simulink model "simulink_431"  (R2024b)
settings: Solver=VariableStepAuto  StartTime=0.0  StopTime=10.0  RelTol=1e-3
values from neighbouring files (symbols this model uses):
  Cvp = cpp * rop * Vp    (= 75000)    [lab1_431.m]    (also in lab2_431.m)
  Cvw = cpp * rop * Vw    (= 300000)    [lab1_431.m]    (also in lab2_431.m)
  dPg = 1000    [lab1_431.m]    (also in lab2_431.m)
  dTzew = 0    [lab1_431.m]    (also in lab2_431.m)
  K1 = heatLossFactor * Kp    (= 240)    [lab1_431.m]    (also in lab2_431.m)
  Kd = Kp * (TwewN - TpN) / (TpN - TzewN)    (= 11.4285714286)    [lab1_431.m]    (also in lab2_431.m)
  Kp = PgN / (TwewN * (heatLossFactor + 1) - heatLossFactor * TzewN - TpN)    (= 80)    [lab1_431.m]    (also in lab2_431.m)
  Pg0 = workPoints(2, i)    [lab1_431.m]    (also in lab2_431.m = 7000)
  stepTime = 500    [lab1_431.m]    (also in lab2_431.m)
  Tzew0 = workPoints(1, i)    [lab1_431.m]    (also in lab2_431.m = -20)
undefined symbols (not defined in the file or in its folder): Tp0, Twew0
settings Model: Creator=maria  LastModifiedBy=maria

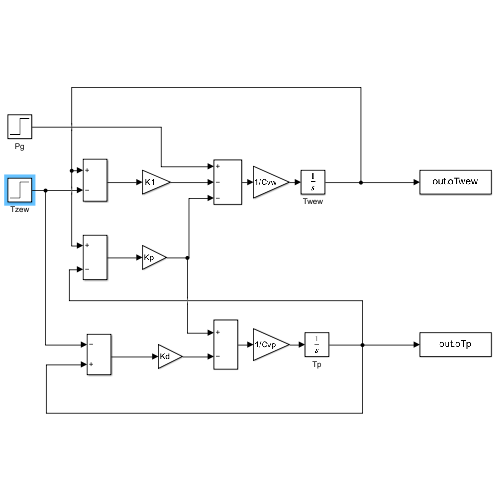
[thumbnail: Simulink's stored preview of the top-level diagram]
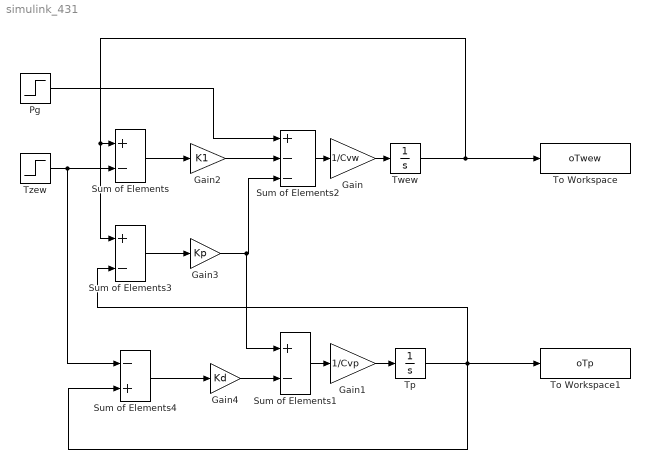
== system simulink_431 ==
  Gain : Gain  Gain=1/Cvw
  Gain1 : Gain  Gain=1/Cvp
  Gain2 : Gain  Gain=K1
  Gain3 : Gain  Gain=Kp
  Gain4 : Gain  Gain=Kd
  Pg : Step  Time=stepTime  Before=Pg0  After=Pg0+dPg  SampleTime=0
  Sum of Elements : Sum  Inputs=+-
  Sum of Elements1 : Sum  Inputs=+-
  Sum of Elements2 : Sum  Inputs=+--
  Sum of Elements3 : Sum  Inputs=+-
  Sum of Elements4 : Sum  Inputs=-+
  To Workspace : ToWorkspace  VariableName=oTwew  SampleTime=-1
  To Workspace1 : ToWorkspace  VariableName=oTp  SampleTime=-1
  Tp : Integrator  InitialCondition=Tp0
  Twew : Integrator  InitialCondition=Twew0
  Tzew : Step  Time=stepTime  Before=Tzew0  After=Tzew0+dTzew  SampleTime=0
  wires:
  Gain1/1 -> Tp/1
  Sum of Elements1/1 -> Gain1/1
  Tzew/1 -> Sum of Elements4/1, Sum of Elements/2
  Twew/1 -> To Workspace/1, Sum of Elements3/1, Sum of Elements/1
  Sum of Elements/1 -> Gain2/1
  Gain2/1 -> Sum of Elements2/2
  Pg/1 -> Sum of Elements2/1
  Tp/1 -> Sum of Elements3/2, Sum of Elements4/2, To Workspace1/1
  Sum of Elements3/1 -> Gain3/1
  Gain3/1 -> Sum of Elements1/1, Sum of Elements2/3
  Sum of Elements2/1 -> Gain/1
  Gain/1 -> Twew/1
  Gain4/1 -> Sum of Elements1/2
  Sum of Elements4/1 -> Gain4/1
